simulink library "INT_SpdDemSwt_VD"  (R2016b)
settings: Solver=VariableStepAuto  StartTime=0.0  StopTime=10.0  RelTol=1e-3
settings Model: Creator=lenovo  LastModifiedBy=lenovo

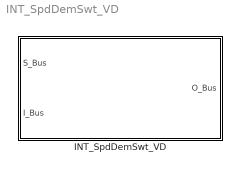
== system INT_SpdDemSwt_VD ==
  INT_SpdDemSwt_VD : Subsystem

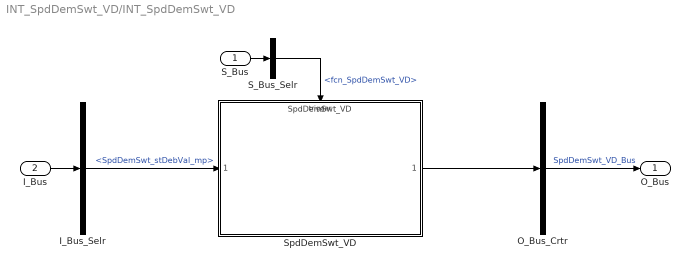
== system INT_SpdDemSwt_VD/INT_SpdDemSwt_VD ==
  S_Bus : Inport
  I_Bus : Inport  Port=2
  I_Bus_Selr : BusSelector  OutputSignals=SpdDemSwt_stDebVal_mp
  O_Bus_Crtr : BusCreator  Inputs=1
  S_Bus_Selr : BusSelector  OutputSignals=fcn_SpdDemSwt_VD
  SpdDemSwt_VD : ModelReference  ModelNameDialog=SpdDemSwt_VD  SimulationMode=Normal  ModelReferenceVersion=1.3  TriggerPortName=function  TriggerPortTriggerType=function-call  TriggerPortStatesWhenEnabling=held
  O_Bus : Outport
  wires:
  S_Bus_Selr/1 -> SpdDemSwt_VD/Trigger  "<fcn_SpdDemSwt_VD>"
  S_Bus/1 -> S_Bus_Selr/1
  I_Bus/1 -> I_Bus_Selr/1
  I_Bus_Selr/1 -> SpdDemSwt_VD/1  "<SpdDemSwt_stDebVal_mp>"
  O_Bus_Crtr/1 -> O_Bus/1  "SpdDemSwt_VD_Bus"
  SpdDemSwt_VD/1 -> O_Bus_Crtr/1
